simulink model "Buck_Converter_Plant_Model"  (R2021a)
settings: Solver=ode15s  StartTime=0.0  StopTime=10  RelTol=1e-3
values from neighbouring files (symbols this model uses):
  C = [0 1]    [Buck_Converter_MPC_Simulation.m]
  L = 400e-6    (= 0.0004)    [Buck_Converter_MPC_Simulation.m]
  Ro = 50    [Buck_Converter_MPC_Simulation.m]
  Vin = 400    [Buck_Converter_MPC_Simulation.m]
settings Model: Creator=byuwono2022  LastModifiedBy=byuwono2022

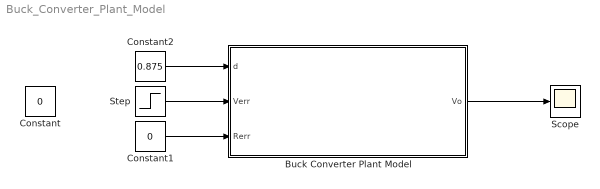
== system Buck_Converter_Plant_Model ==
  Buck Converter Plant Model : Subsystem
  Constant : Constant  Value=0
  Constant1 : Constant  Value=0
  Constant2 : Constant  Value=0.875
  Scope : Scope
  Step : Step  Time=6  After=0.05  SampleTime=0
  wires:
  Constant1/1 -> Buck Converter Plant Model/3(Rerr)
  Constant2/1 -> Buck Converter Plant Model/1(d)
  Buck Converter Plant Model/1(Vo) -> Scope/1
  Step/1 -> Buck Converter Plant Model/2(Verr)

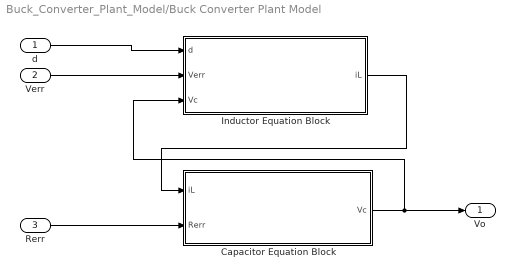
== system Buck_Converter_Plant_Model/Buck Converter Plant Model ==
  d : Inport
  Verr : Inport  Port=2
  Rerr : Inport  Port=3
  Capacitor Equation Block : Subsystem
  Inductor Equation Block : Subsystem
  Vo : Outport
  wires:
  Inductor Equation Block/1(iL) -> Capacitor Equation Block/1(iL)
  Capacitor Equation Block/1(Vc) -> Vo/1, Inductor Equation Block/3(Vc)
  Verr/1 -> Inductor Equation Block/2(Verr)
  Rerr/1 -> Capacitor Equation Block/2(Rerr)
  d/1 -> Inductor Equation Block/1(d)

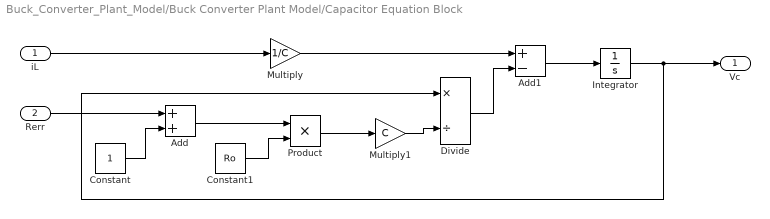
== system Buck_Converter_Plant_Model/Buck Converter Plant Model/Capacitor Equation Block ==
  iL : Inport
  Rerr : Inport  Port=2
  Add : Sum
  Add1 : Sum  Inputs=+-
  Constant : Constant
  Constant1 : Constant  Value=Ro
  Divide : Product  Inputs=*/
  Integrator : Integrator  InitialCondition=0.0000000001
  Multiply : Gain  Gain=1/C
  Multiply1 : Gain  Gain=C
  Product : Product
  Vc : Outport
  wires:
  Integrator/1 -> Vc/1, Divide/1
  iL/1 -> Multiply/1
  Multiply1/1 -> Divide/2
  Constant/1 -> Add/2
  Rerr/1 -> Add/1
  Add1/1 -> Integrator/1
  Add/1 -> Product/1
  Constant1/1 -> Product/2
  Product/1 -> Multiply1/1
  Divide/1 -> Add1/2
  Multiply/1 -> Add1/1

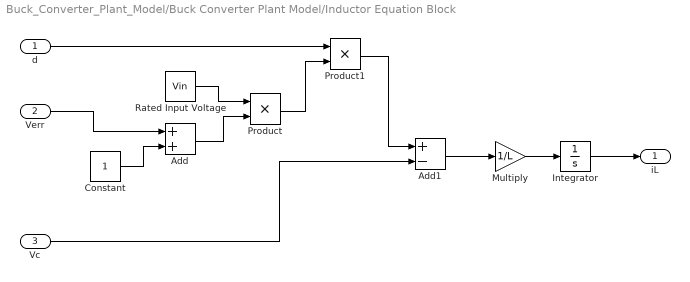
== system Buck_Converter_Plant_Model/Buck Converter Plant Model/Inductor Equation Block ==
  d : Inport
  Verr : Inport  Port=2
  Vc : Inport  Port=3
  Add : Sum
  Add1 : Sum  Inputs=+-
  Constant : Constant
  Integrator : Integrator  InitialCondition=0.0000000001
  Multiply : Gain  Gain=1/L
  Product : Product
  Product1 : Product
  Rated Input Voltage : Constant  Value=Vin
  iL : Outport
  wires:
  Multiply/1 -> Integrator/1
  Vc/1 -> Add1/2
  Product/1 -> Product1/2
  Add/1 -> Product/2
  Integrator/1 -> iL/1
  Verr/1 -> Add/1
  Product1/1 -> Add1/1
  d/1 -> Product1/1
  Add1/1 -> Multiply/1
  Constant/1 -> Add/2
  Rated Input Voltage/1 -> Product/1
